simulink model "Sub3_2023"  (R2023b)
settings: Solver=FixedStepDiscrete  StartTime=0.0  StopTime=4.5  FixedStep=75e-6  RelTol=1e-3  EnableMultiTasking=on
undefined symbols (not defined in the file or in its folder): D1, D11, Delta
libraries: spsSeriesRLCBranchLib x41, spsLoadFlowBusLib x29, spsDistributedParametersLineLib x19, spsThreePhaseSeriesRLCLoadLib x15, spsThreePhaseTransformerTwoWindingsLib x13, spsThreePhaseParallelRLCLoadLib x11, spsThreePhaseVIMeasurementLib x11, spsSynchronousMachinepuStandardLib x7, spsExcitationSystemLib x7, spsHydraulicTurbineandGovernorLib x7, spsGenericPowerSystemStabilizerLib x7, spsMultiBandPowerSystemStabilizerLib x7
(part 2 of 5)

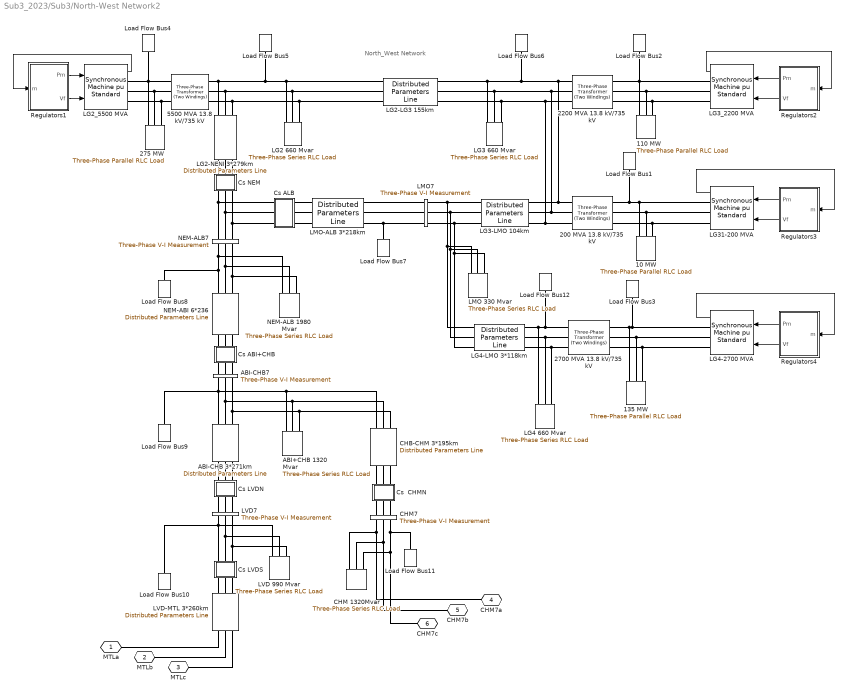
== system Sub3_2023/Sub3/North-West Network2 ==
  note: North_West Network
  10 MW : spsThreePhaseParallelRLCLoadLib/Three-Phase Parallel RLC Load  LConnTagsString=A|B|C  Configuration=Y (grounded)  NominalVoltage=(13800)*1  Vabc=[1e3 1e3 1e3]  Vabcp=[1e3 1e3 1e3]  NominalFrequency=60  UnbalancedPower=off  ActivePower=10000000  InductivePower=0  CapacitivePower=0  Pabc=[10e3 9e3 11e3]  QLabc=[100 90 110]  QCabc=[100 90 110]  Pabcp=[10e3 9e3 11e3]  QLabcp=[100 90 110]  QCabcp=[100 90 110]  Measurements=None  LoadType=constant PQ
  110 MW : spsThreePhaseParallelRLCLoadLib/Three-Phase Parallel RLC Load  LConnTagsString=A|B|C  Configuration=Y (grounded)  NominalVoltage=(13800)*1  Vabc=[1e3 1e3 1e3]  Vabcp=[1e3 1e3 1e3]  NominalFrequency=60  UnbalancedPower=off  ActivePower=110000000  InductivePower=0  CapacitivePower=0  Pabc=[10e3 9e3 11e3]  QLabc=[100 90 110]  QCabc=[100 90 110]  Pabcp=[10e3 9e3 11e3]  QLabcp=[100 90 110]  QCabcp=[100 90 110]  Measurements=None  LoadType=constant PQ
  135 MW : spsThreePhaseParallelRLCLoadLib/Three-Phase Parallel RLC Load  LConnTagsString=A|B|C  Configuration=Y (grounded)  NominalVoltage=(13800)*1  Vabc=[1e3 1e3 1e3]  Vabcp=[1e3 1e3 1e3]  NominalFrequency=60  UnbalancedPower=off  ActivePower=135000000  InductivePower=0  CapacitivePower=0  Pabc=[10e3 9e3 11e3]  QLabc=[100 90 110]  QCabc=[100 90 110]  Pabcp=[10e3 9e3 11e3]  QLabcp=[100 90 110]  QCabcp=[100 90 110]  Measurements=None  LoadType=constant PQ
  200 MVA 13.8 kV/735 kV : spsThreePhaseTransformerTwoWindingsLib/Three-Phase Transformer (Two Windings)  Winding1Connection=Delta (D1)  Winding2Connection=Yg  CoreType=Three single-phase transformers  SetSaturation=off  Hysteresis=off  DataFile='basic_model'  SetInitialFlux=off  Measurements=None  UNITS=pu  NominalPower=[ 200e6 60 ]  Winding1="[ 13.8e3 0.002  0.0]"  Winding2=[ 735e3 0.002 0.12]  Rm=500  Lm=500  L0=0.5  Saturation="[ 0,0  ;  0.005,1.2  ;  1.0,1.4 ]"  InitialFluxes=[ 0.8 , -0.8 , 0.7 ]  BreakLoop=off  DiscreteSolver=Trapezoidal iterative  DataType=off  TransfoNumber=0
  2200 MVA 13.8 kV/735 kV : spsThreePhaseTransformerTwoWindingsLib/Three-Phase Transformer (Two Windings)  Winding1Connection=Delta (D1)  Winding2Connection=Yg  CoreType=Three single-phase transformers  SetSaturation=off  Hysteresis=off  DataFile='basic_model'  SetInitialFlux=off  Measurements=None  UNITS=pu  NominalPower=[ 2200e6 60 ]  Winding1="[ 13.8e3 0.002  0.0]"  Winding2=[ 735e3 0.002 0.12]  Rm=500  Lm=500  L0=0.5  Saturation="[ 0,0  ;  0.005,1.2  ;  1.0,1.4 ]"  InitialFluxes=[ 0.8 , -0.8 , 0.7 ]  BreakLoop=off  DiscreteSolver=Trapezoidal iterative  DataType=off  TransfoNumber=0
  2700 MVA 13.8 kV/735 kV : spsThreePhaseTransformerTwoWindingsLib/Three-Phase Transformer (Two Windings)  Winding1Connection=Delta (D1)  Winding2Connection=Yg  CoreType=Three single-phase transformers  SetSaturation=off  Hysteresis=off  DataFile='basic_model'  SetInitialFlux=off  Measurements=None  UNITS=pu  NominalPower=[ 2700e6 60 ]  Winding1="[ 13.8e3 0.002  0.0]"  Winding2=[ 735e3 0.002 0.12]  Rm=500  Lm=500  L0=0.5  Saturation="[ 0,0  ;  0.005,1.2  ;  1.0,1.4 ]"  InitialFluxes=[ 0.8 , -0.8 , 0.7 ]  BreakLoop=off  DiscreteSolver=Trapezoidal iterative  DataType=off  TransfoNumber=0
  275 MW : spsThreePhaseParallelRLCLoadLib/Three-Phase Parallel RLC Load  LConnTagsString=A|B|C  Configuration=Y (grounded)  NominalVoltage=(13800)*1  Vabc=[1e3 1e3 1e3]  Vabcp=[1e3 1e3 1e3]  NominalFrequency=60  UnbalancedPower=off  ActivePower=275000000  InductivePower=0  CapacitivePower=0  Pabc=[10e3 9e3 11e3]  QLabc=[100 90 110]  QCabc=[100 90 110]  Pabcp=[10e3 9e3 11e3]  QLabcp=[100 90 110]  QCabcp=[100 90 110]  Measurements=None  LoadType=constant PQ
  5500 MVA 13.8 kV/735 kV : spsThreePhaseTransformerTwoWindingsLib/Three-Phase Transformer (Two Windings)  Winding1Connection=Delta (D1)  Winding2Connection=Yg  CoreType=Three single-phase transformers  SetSaturation=off  Hysteresis=off  DataFile='basic_model'  SetInitialFlux=off  Measurements=None  UNITS=pu  NominalPower=[ 5500e6 60 ]  Winding1="[ 13.8e3 0.002  0.0]"  Winding2=[ 735e3 0.002 0.12]  Rm=500  Lm=500  L0=0.5  Saturation="[ 0,0  ;  0.005,1.2  ;  1.0,1.4 ]"  InitialFluxes=[ 0.8 , -0.8 , 0.7 ]  BreakLoop=off  DiscreteSolver=Trapezoidal iterative  DataType=off  TransfoNumber=0
  ABI+CHB 1320 Mvar : spsThreePhaseSeriesRLCLoadLib/Three-Phase Series RLC Load  LConnTagsString=A|B|C  Configuration=Y (grounded)  NominalVoltage=735e3  Vabc=[1e3 1e3 1e3]  Vabcp=[1e3 1e3 1e3]  NominalFrequency=60  UnbalancedPower=off  ActivePower=4400000  InductivePower=1320e6  CapacitivePower=0  Pabc=[10e3 9e3 11e3]  QLabc=[100 90 110]  QCabc=[100 90 110]  Pabcp=[10e3 9e3 11e3]  QLabcp=[100 90 110]  QCabcp=[100 90 110]  Measurements=None  LoadType=constant Z
  ABI-CHB 3*271km : spsDistributedParametersLineLib/Distributed Parameters Line  Phases=3  Length=271  Frequency=60  Resistance="[0.01273  0.3864]/3"  Inductance="[0.9337e-3  4.1264e-3]/3"  Capacitance=[12.74e-9 7.751e-9]*3  x1=[-0.001575 2.82252813868878e-08 -103484.456536265 -819305.847115468;-0.0015 2.83466164414192e-08 -80280.8596539526 -821903.919579529;-0.001425 2.84452916444852e-08 -57013.087480771 -823844.97462583;-0.00135 2.85212281166381e-08 -33699.7399177867 -825127.460604666;-0.001275 2.8574365155424e-08 -10359.4532983355 -825750.352316369;-0.0012 2.86046602839071e-08 12989.1145095774 -825713.151830833;-0.001125 2.86120892846252e-08 36327.2990180915 -825015.888885559;-0.00105 2.85966462189488e-08 59636.4440395969 -823659.120861876;-0.000975 2.85583434318284e-08 82897.9166002052 -821643.932339383;-0.0009 2.84972115419259e-08 106093.121834664 -818971.934228952;-0.000825 2.84132994171387e-08 129203.517850807 -815645.262484989;-0.00075 2.83066741355355e-08 152210.630551661 -811666.576397987;-0.000675 2.8177420931735e-08 175096.068403352 -807039.056468727;-0.0006 2.80256431287707e-08 197841.537137021 -801766.401865838;-0.000525 2.78514620554959e-08 220428.85437298 -795852.827468734;-0.00045 2.76550169495957e-08 242839.964155428 -789303.060498309;-0.000375 2.74364648462819e-08 265056.951386106 -782122.336738063;-0.0003 2.71959804527619e-08 287062.056145353 -774316.396348701;-0.000225 2.69337560085805e-08 308837.687889115 -765891.479279537;-0.00015 2.66500011319461e-08 330366.439510553 -756854.320280369;-7.5e-05 2.63449426521655e-08 351631.101255022 -747212.143517828]  x2=[-0.001575 6.39967509370556e-08 -329701.158011639 -748762.18711566;-0.0015 6.42027184101767e-08 -308401.44101005 -757783.743021151;-0.001425 6.43573632125353e-08 -286855.192615217 -766199.538196952;-0.00135 6.44605617234425e-08 -265079.63656844 -774002.845185164;-0.001275 6.45122314475876e-08 -243092.179916044 -781187.426141576;-0.0012 6.45123310809837e-08 -220910.399094458 -787747.537822099;-0.001125 6.44608605439855e-08 -198552.025879879 -793677.936173828;-0.00105 6.43578609813526e-08 -176034.933213759 -798973.88052706;-0.000975 6.42034147293596e-08 -153377.120915453 -803631.137384908;-0.0009 6.3997645249977e-08 -130596.701293435 -807645.9838075;-0.000825 6.37407170321785e-08 -107711.884666601 -811015.210388034;-0.00075 6.34328354604501e-08 -84740.9648072106 -813736.123818332;-0.000675 6.30742466506096e-08 -61702.3043171338 -815806.549041831;-0.0006 6.26652372530649e-08 -38614.3199490629 -817224.830992284;-0.000525 6.22061342236703e-08 -15495.4678844435 -817989.835916801;-0.00045 6.16973045623632e-08 7635.77102011404 -818100.95228215;-0.000375 6.11391550197893e-08 30760.9060061493 -817558.09126361;-0.0003 6.0532131772153e-08 53861.451194581 -816361.686815971;-0.000225 5.98767200645508e-08 76918.9403630354 -814512.695326645;-0.00015 5.91734438230734e-08 99914.941707463 -812012.594851136;-7.5e-05 5.8422865235988e-08 122831.07257624 -808863.383931513]  x3=[-0.001575 1.3106440852015e-10 -747.841433918081 -1501.46113433883;-0.0015 1.39263740651287e-10 -705.09503694866 -1522.00231179706;-0.001425 1.47351747478955e-10 -661.784997795018 -1541.32682389466;-0.00135 1.55321963574244e-10 -617.945937839789 -1559.41922291233;-0.001275 1.63168017668359e-10 -573.612901356741 -1576.26504606312;-0.0012 1.70883637745703e-10 -528.82132749692 -1591.85082705374;-0.001125 1.78462656057641e-10 -483.607021959136 -1606.16410684936;-0.00105 1.85899014052897e-10 -438.006128367433 -1619.19344363309;-0.000975 1.93186767220669e-10 -392.055099378431 -1630.92842195248;-0.0009 2.00320089842582e-10 -345.790667541631 -1641.35966104539;-0.000825 2.07293279649674e-10 -299.249815935972 -1650.47882233891;-0.00075 2.14100762380708e-10 -252.46974860613 -1658.27861611503;-0.000675 2.20737096238147e-10 -205.487860822169 -1664.75280733794;-0.0006 2.27196976238244e-10 -158.341709186337 -1669.89622063824;-0.000525 2.33475238451766e-10 -111.06898161089 -1673.70474445002;-0.00045 2.3956686413196e-10 -63.7074671909556 -1676.17533429764;-0.000375 2.45466983726464e-10 -16.2950259965059 -1677.30601522935;-0.0003 2.51170880769947e-10 31.1304411924031 -1677.09588339614;-0.000225 2.56673995654386e-10 78.5310231829346 -1675.54510677417;-0.00015 2.61971929273943e-10 125.868828675099 -1672.65492503054;-7.5e-05 2.67060446541544e-10 173.106016551477 -1668.42764853232]  x4=[-0.001575 1.93458409580896e-10 -7080.29438162651 -14859.1258761624;-0.0015 1.8934224315803e-10 -6657.38891400317 -15053.3510061728;-0.001425 1.85074719443017e-10 -6229.16163154343 -15235.5427177129;-0.00135 1.80659249829019e-10 -5795.95485258481 -15405.5553695161;-0.001275 1.76099363974887e-10 -5358.11487599811 -15563.2530560699;-0.0012 1.71398706983604e-10 -4915.99170436145 -15708.5097162563;-0.001125 1.66561036488447e-10 -4469.93876417352 -15841.2092341238;-0.00105 1.6159021964919e-10 -4020.31262332986 -15961.2455317082;-0.000975 1.56490230060759e-10 -3567.47270608796 -16068.5226538298;-0.0009 1.51265144576798e-10 -3111.78100574897 -16162.9548447986;-0.000825 1.45919140050696e-10 -2653.60179528584 -16244.4666169659;-0.00075 1.40456489996676e-10 -2193.30133614902 -16312.9928110683;-0.000675 1.34881561173609e-10 -1731.24758548272 -16368.4786483147;-0.0006 1.29198810094297e-10 -1267.80990198557 -16410.8797741758;-0.000525 1.23412779463003e-10 -803.358750650903 -16440.1622938402;-0.00045 1.17528094544086e-10 -338.265406622771 -16456.3027993099;-0.000375 1.1154945946463e-10 127.098341595781 -16459.2883881117;-0.0003 1.05481653454042e-10 592.360489344731 -16449.1166736116;-0.000225 9.93295270236066e-11 1057.14911318192 -16425.7957869225;-0.00015 9.30979980890611e-11 1521.09266819295 -16389.3443704045;-7.5e-05 8.67920480392902e-11 1983.82028499853 -16339.7915627621]  x5=0.00153261764655846  V1=ones(3,3)  V2=ones(3,3)  I1=ones(3,3)  I2=ones(3,3)  nHarmo=1  Measurements=None  Decoupling=on  VsMag0=[674275.598206265 674275.04688371 674275.387112359]  VrMag0=[668005.988427177 668005.867389108 668005.726368268]  VsAngle0=[-3.17875639506823 -123.17875005978 116.821287344135]  VrAngle0=[-19.7452308032682 -139.745250763836 100.254768207184]  IsMag0=[1378.35069563023 1378.34088888681 1378.33344706177]  IrMag0=[13525.2461163751 13525.2482026069 13525.2572474099]  IsAngle0=[-22.4561903613039 -142.456782921015 97.5438663997709]  IrAngle0=[-21.4575985540813 -141.457549208484 98.5424184650414]
      settings: AttributesFormatString=\n  LibrarySourceBlock=sps_lib/Power Grid Elements/Distributed Parameters Line
  ABI-CHB7 : spsThreePhaseVIMeasurementLib/Three-Phase V-I Measurement  VoltageMeasurement=no  SetLabelV=on  LabelV=Vabc_ABI7  Vpu=on  VpuLL=off  CurrentMeasurement=no  SetLabelI=off  LabelI=A1  Ipu=off  Pbase=100e6  Vbase=500e3  OutputType=Magnitude  PhasorSimulation=off  PSBequivalent=0
  CHB-CHM 3*195km : spsDistributedParametersLineLib/Distributed Parameters Line  Phases=3  Length=195  Frequency=60  Resistance="[0.01273  0.3864]/3"  Inductance="[0.9337e-3  4.1264e-3]/3"  Capacitance=[12.74e-9 7.751e-9]*3  x1=[-0.001125 2.86120892846252e-08 0 0;-0.00105 2.85966462189488e-08 0 0;-0.000975 2.85583434318284e-08 0 0;-0.0009 2.84972115419259e-08 0 0;-0.000825 2.84132994171387e-08 0 0;-0.00075 2.83066741355355e-08 0 0;-0.000675 2.8177420931735e-08 175096.068403352 -807039.056468727;-0.0006 2.80256431287707e-08 197841.537137021 -801766.401865838;-0.000525 2.78514620554959e-08 220428.85437298 -795852.827468734;-0.00045 2.76550169495957e-08 242839.964155428 -789303.060498309;-0.000375 2.74364648462819e-08 265056.951386106 -782122.336738063;-0.0003 2.71959804527619e-08 287062.056145353 -774316.396348701;-0.000225 2.69337560085805e-08 308837.687889115 -765891.479279537;-0.00015 2.66500011319461e-08 330366.439510553 -756854.320280369;-7.5e-05 2.63449426521655e-08 351631.101255022 -747212.143517828]  x2=[-0.001125 1.92257365142825e-08 0 0;-0.00105 1.91619388673599e-08 0 0;-0.000975 1.90828234596942e-08 0 0;-0.0009 1.89884535349318e-08 0 0;-0.000825 1.88789045309467e-08 0 0;-0.00075 1.87542640195364e-08 0 0;-0.000675 1.86146316364188e-08 86661.6913680594 -814290.344127245;-0.0006 1.84601190015845e-08 109647.510746625 -811514.902082648;-0.000525 1.82908496300696e-08 132545.679582764 -808090.74744192;-0.00045 1.81069588332198e-08 155337.893430661 -804020.61742189;-0.000375 1.79085936105245e-08 178005.932543298 -799307.765622221;-0.0003 1.76959125321075e-08 200531.676437043 -793955.959424533;-0.000225 1.7469085611969e-08 222897.118376882 -787969.476980814;-0.00015 1.72282941720782e-08 245084.37977073 -781353.103793534;-7.5e-05 1.69737306974281e-08 267075.724461307 -774112.128890185]  x3=[-0.001125 1.04687394448767e-10 0 0;-0.00105 1.02659720732973e-10 0 0;-0.000975 1.00549982407171e-10 0 0;-0.0009 9.83598659638991e-11 0 0;-0.000825 9.60911221487322e-11 0 0;-0.00075 9.37455645607631e-11 0 0;-0.000675 9.13250682028394e-11 335.259499975967 -5255.1630322511;-0.0006 8.88315679827147e-11 483.692851575627 -5243.58412650791;-0.000525 8.62670571663132e-11 631.739546510486 -5227.81357984352;-0.00045 8.36335857843431e-11 779.281238517804 -5207.86399899163;-0.000375 8.09332589935339e-11 926.199985026453 -5183.75133134194;-0.0003 7.81682353938056e-11 1072.37834143841 -5155.49485219203;-0.000225 7.53407253027176e-11 1217.69945501215 -5123.11714933899;-0.00015 7.24529889885743e-11 1362.04715827299 -5086.64410502309;-7.5e-05 6.95073348636015e-11 1505.30606187552 -5046.10487523791]  x4=[-0.001125 8.04385281148192e-11 0 0;-0.00105 8.32616576275703e-11 0 0;-0.000975 8.601822904516e-11 0 0;-0.0009 8.8706038806574e-11 0 0;-0.000825 9.1322938317814e-11 0 0;-0.00075 9.38668356694505e-11 0 0;-0.000675 9.63356973088636e-11 265.942029612726 -12956.0177279482;-0.0006 9.87275496658336e-11 632.108856780154 -12943.3211843337;-0.000525 1.01040480730183e-10 997.770385799061 -12920.277947804;-0.00045 1.03272641580208e-10 1362.63431243796 -12886.9064387697;-0.000375 1.05422247860678e-10 1726.4089700565 -12843.2333339044;-0.0003 1.07487581209222e-10 2088.80356275932 -12789.2935448202;-0.000225 1.09466990629963e-10 2449.52839785384 -12725.1301901589;-0.00015 1.11358893813296e-10 2808.29511742615 -12650.7945611247;-7.5e-05 1.13161778400763e-10 3164.81692884995 -12566.3460804819]  x5=0.0011028060556417  V1=ones(3,3)  V2=ones(3,3)  I1=ones(3,3)  I2=ones(3,3)  nHarmo=1  Measurements=None  Decoupling=on  VsMag0=[674275.598206265 674275.04688371 674275.387112359]  VrMag0=[668620.174918554 668620.122023149 668619.982355037]  VsAngle0=[-3.17875639506823 -123.17875005978 116.821287344135]  VrAngle0=[-9.34509688682244 -129.345113323862 110.65489882013]  IsMag0=[4319.32992808175 4319.31639781994 4319.30396194623]  IrMag0=[10629.372791075 10629.3784873068 10629.3938662882]  IsAngle0=[-11.7695166369384 -131.769810740508 108.230491745392]  IrAngle0=[-14.2441447349322 -134.244031285624 105.755885398874]
      settings: AttributesFormatString=\n  LibrarySourceBlock=sps_lib/Power Grid Elements/Distributed Parameters Line
  CHM 1320Mvar : spsThreePhaseSeriesRLCLoadLib/Three-Phase Series RLC Load  LConnTagsString=A|B|C  Configuration=Y (grounded)  NominalVoltage=735e3  Vabc=[1e3 1e3 1e3]  Vabcp=[1e3 1e3 1e3]  NominalFrequency=60  UnbalancedPower=off  ActivePower=4400000  InductivePower=1320e6  CapacitivePower=0  Pabc=[10e3 9e3 11e3]  QLabc=[100 90 110]  QCabc=[100 90 110]  Pabcp=[10e3 9e3 11e3]  QLabcp=[100 90 110]  QCabcp=[100 90 110]  Measurements=None  LoadType=constant Z
  CHM7 : spsThreePhaseVIMeasurementLib/Three-Phase V-I Measurement  VoltageMeasurement=no  SetLabelV=on  LabelV=Vabc_CHM7  Vpu=on  VpuLL=off  CurrentMeasurement=no  SetLabelI=off  LabelI=A1  Ipu=off  Pbase=100e6  Vbase=735e3  OutputType=Magnitude  PhasorSimulation=off  PSBequivalent=0
  "Cs  CHMN " : Subsystem  mask{Xc=25/3}
      mask prompts: Xc "Condensator Reactance at  60Hz  (ohm):"
      mask help: Series Compensation
      mask init:
      | Cs=1/Xc/(2*pi*60);
      mask Display: disp('Cs')
  "Cs ABI+CHB " : Subsystem  mask{Xc=25/6}
      mask prompts: Xc "Condensator Reactance at  60Hz  (ohm):"
      mask help: Series Compensation
      mask init:
      | Cs=1/Xc/(2*pi*60);
      mask Display: disp('Cs')
  Cs ALB : Subsystem  mask{Xc=16/3}
      mask prompts: Xc "Reactance @ 60Hz du condensateur (ohm):"
      mask init:
      | Cs=1/Xc/(2*pi*60);
      mask Display: disp('Cs')
  "Cs LVDN " : Subsystem  mask{Xc=34/3}
      mask prompts: Xc "Condensator Reactance at  60Hz  (ohm):"
      mask help: Series Compensation
      mask init:
      | Cs=1/Xc/(2*pi*60);
      mask Display: disp('Cs')
  "Cs LVDS " : Subsystem  mask{Xc=34/3}
      mask prompts: Xc "Condensator Reactance at  60Hz  (ohm):"
      mask help: Series Compensation
      mask init:
      | Cs=1/Xc/(2*pi*60);
      mask Display: disp('Cs')
  "Cs NEM " : Subsystem  mask{Xc=16/3}
      mask prompts: Xc "Condensator Reactance at  60Hz  (ohm):"
      mask help: Series Compensation
      mask init:
      | Cs=1/Xc/(2*pi*60);
      mask Display: disp('Cs')
  LG2 660 Mvar : spsThreePhaseSeriesRLCLoadLib/Three-Phase Series RLC Load  LConnTagsString=A|B|C  Configuration=Y (grounded)  NominalVoltage=735e3  Vabc=[1e3 1e3 1e3]  Vabcp=[1e3 1e3 1e3]  NominalFrequency=60  UnbalancedPower=off  ActivePower=2200000  InductivePower=660e6  CapacitivePower=0  Pabc=[10e3 9e3 11e3]  QLabc=[100 90 110]  QCabc=[100 90 110]  Pabcp=[10e3 9e3 11e3]  QLabcp=[100 90 110]  QCabcp=[100 90 110]  Measurements=None  LoadType=constant Z
  LG2-LG3 155km : spsDistributedParametersLineLib/Distributed Parameters Line  Phases=3  Length=155  Frequency=60  Resistance="[0.01273  0.3864]"  Inductance="[0.9337e-3  4.1264e-3]"  Capacitance=[12.74e-9 7.751e-9]  x1=[-0.0009 5.26292056031291e-10 371984.24988172 -674633.962928139;-0.000825 5.67978956510661e-10 390907.83551166 -663848.049238456;-0.00075 6.09211823302567e-10 409518.935398982 -652531.465575427;-0.000675 6.49957695484177e-10 427802.672115196 -640693.258242884;-0.0006 6.90184001428704e-10 445744.429920922 -628342.890522636;-0.000525 7.29858584842658e-10 463329.866449487 -615490.235109674;-0.00045 7.689497304711e-10 480544.924171997 -602145.566220082;-0.000375 8.07426189450328e-10 497375.841634708 -588319.551377989;-0.0003 8.45257204287745e-10 513809.164459722 -574023.242888115;-0.000225 8.82412533448924e-10 529831.75610021 -559268.069000727;-0.00015 9.18862475532227e-10 545430.80834157 -544065.824776068;-7.5e-05 9.54577893011657e-10 560593.851540113 -528428.66265557]  x2=[-0.0009 -2.84133647185834e-10 375373.731714329 -666225.896356635;-0.000825 -3.30481312850429e-10 394058.262242269 -655347.523812927;-0.00075 -3.76564796810066e-10 412427.788624667 -643945.276485836;-0.000675 -4.22347260632767e-10 430467.626543196 -632028.269157416;-0.0006 -4.67792106517448e-10 448163.355227441 -619606.028100988;-0.000525 -5.12863006549638e-10 465500.828982646 -606688.483465986;-0.00045 -5.5752393174146e-10 482466.188497565 -593285.961339946;-0.000375 -6.0173918083265e-10 499045.871923379 -579409.175493991;-0.0003 -6.454734088296e-10 515226.625714835 -565069.218818404;-0.000225 -6.88691655259606e-10 530995.515224926 -550277.554455142;-0.00015 -7.31359372117733e-10 546339.93504465 -535046.006634378;-7.5e-05 -7.73442451483964e-10 561247.619079581 -519386.751222389]  x3=[-0.0009 1.24259718768771e-11 1272.11889165543 -2673.50704029682;-0.000825 1.22505792748699e-11 1347.19195646242 -2636.47471081189;-0.00075 1.20653937472306e-11 1421.18809663214 -2597.33482378256;-0.000675 1.18705633284365e-11 1494.04816078233 -2556.11866703565;-0.0006 1.16662437629433e-11 1565.71390569248 -2512.85918813624;-0.000525 1.14525983806856e-11 1636.12804286265 -2467.59096804986;-0.00045 1.12297979665129e-11 1705.23428430896 -2420.35019349904;-0.000375 1.09980206236675e-11 1772.97738755935 -2371.17462803613;-0.0003 1.07574516314109e-11 1839.30319981359 -2320.10358185576;-0.000225 1.05082832969147e-11 1904.15870123218 -2267.17788037083;-0.00015 1.02507148015331e-11 1967.49204731961 -2212.43983157731;-7.5e-05 9.98495204158025e-12 2029.25261036805 -2155.9331922339]  x4=[-0.0009 -1.18025559648927e-11 974.452643997273 -2530.47846704078;-0.000825 -1.16866166993846e-11 1045.60107405565 -2501.91852232173;-0.00075 -1.15613353312983e-11 1115.91366661366 -2471.35858221657;-0.000675 -1.14268120086425e-11 1185.33421486063 -2438.82307587384;-0.0006 -1.1283154267303e-11 1253.80722507246 -2404.3380116795;-0.000525 -1.11304769450804e-11 1321.27796097246 -2367.93095646624;-0.00045 -1.09689020898898e-11 1387.69248748669 -2329.63101347693;-0.000375 -1.07985588621984e-11 1452.99771385883 -2289.4687991;-0.0003 -1.06195834317761e-11 1517.14143609013 -2247.47641839511;-0.000225 -1.04321188688434e-11 1580.07237867045 -2203.6874394289;-0.00015 -1.02363150297038e-11 1641.74023556719 -2158.13686644117;-7.5e-05 -1.00323284369503e-11 1702.09571043908 -2110.86111186299]  x5=0.000876589428843401  V1=ones(3,3)  V2=ones(3,3)  I1=ones(3,3)  I2=ones(3,3)  nHarmo=1  Measurements=None  Decoupling=on  VsMag0=[629022.539261878 629021.416248132 629022.998971626]  VrMag0=[624373.329666333 624372.279031978 624373.793132847]  VsAngle0=[18.311762016023 -101.68813057419 138.311904308239]  VrAngle0=[18.8383509464139 -101.161544280644 138.838486827789]  IsMag0=[2426.2546778534 2426.24994282991 2426.25518358254]  IrMag0=[2222.110354709 2222.10693756313 2222.11326012476]  IsAngle0=[14.8862320606581 -105.113689591392 134.886368071059]  IrAngle0=[10.5010096554468 -109.498852970977 130.501154646759]
      settings: AttributesFormatString=\n  LibrarySourceBlock=sps_lib/Power Grid Elements/Distributed Parameters Line
  LG2-NENI 3*279km : spsDistributedParametersLineLib/Distributed Parameters Line  Phases=3  Length=279  Frequency=60  Resistance="[0.01273  0.3864]/3"  Inductance="[0.9337e-3  4.1264e-3]/3"  Capacitance=[12.74e-9 7.751e-9]*3  x1=[-0.00165 9.19274009253425e-11 168997.444323809 -751627.644710141;-0.001575 1.36275318057477e-10 190178.800706863 -746549.517209721;-0.0015 1.80514298785439e-10 211208.131066464 -740874.609447834;-0.001425 2.24608979144913e-10 232068.624877684 -734607.457858916;-0.00135 2.68524110523091e-10 252743.606580946 -727753.072308057;-0.001275 3.12224587835874e-10 273216.548912214 -720316.932086191;-0.0012 3.55675477590337e-10 293471.086114634 -712304.981530033;-0.001125 3.98842045810032e-10 313491.027021073 -703723.625270272;-0.00105 4.41689785800794e-10 333260.367997085 -694579.723111802;-0.000975 4.84184445734868e-10 352763.305733975 -684880.584550103;-0.0009 5.26292056031291e-10 371984.24988172 -674633.962928139;-0.000825 5.67978956510661e-10 390907.83551166 -663848.049238455;-0.00075 6.09211823302567e-10 409518.935398982 -652531.465575427;-0.000675 6.49957695484177e-10 427802.672115196 -640693.258242883;-0.0006 6.90184001428704e-10 445744.429920922 -628342.890522636;-0.000525 7.29858584842658e-10 463329.866449487 -615490.235109674;-0.00045 7.689497304711e-10 480544.924171997 -602145.566220082;-0.000375 8.07426189450328e-10 497375.841634708 -588319.551377989;-0.0003 8.45257204287745e-10 513809.164459722 -574023.242888115;-0.000225 8.82412533448924e-10 529831.75610021 -559268.069000727;-0.00015 9.18862475532227e-10 545430.80834157 -544065.824776068;-7.5e-05 9.54577893011657e-10 560593.851540113 -528428.66265557]  x2=[-0.00165 1.62069086814666e-08 -47534.306464813 -809002.98310623;-0.001575 1.62900091845941e-08 -24644.3461225884 -810023.426229766;-0.0015 1.63600877036248e-08 -1734.68546714459 -810396.349020148;-0.001425 1.64170882188631e-08 21176.36186932 -810121.453368603;-0.00135 1.6460965164969e-08 44070.4811461156 -809198.95902251;-0.001275 1.64916834673833e-08 66929.3711545839 -807629.603409733;-0.0012 1.6509218570365e-08 89734.7588478049 -805414.641049137;-0.001125 1.6513556456621e-08 112468.413947791 -802555.842547744;-0.00105 1.65046936585115e-08 135112.163518491 -799055.493185335;-0.000975 1.64826372608217e-08 157647.906492961 -794916.391087632;-0.0009 1.64474048950984e-08 180057.628143073 -790141.844989523;-0.000825 1.63990247255557e-08 202323.414480223 -784735.671590104;-0.00075 1.63375354265608e-08 224427.466575488 -778702.192501675;-0.000675 1.62629861517186e-08 246352.114787829 -772046.230795103;-0.0006 1.61754364945788e-08 268079.832888922 -764773.107144337;-0.000525 1.60749564409977e-08 289593.252073363 -756888.63557314;-0.00045 1.59616263131928e-08 310875.174843021 -748399.118807451;-0.000375 1.58355367055341e-08 331908.58875446 -739311.343237078;-0.0003 1.56967884121249e-08 352676.68001842 -729632.573490764;-0.000225 1.5545492346228e-08 373162.846940507 -719370.546628954;-0.00015 1.53817694516034e-08 393350.713192334 -708533.465958907;-7.5e-05 1.52057506058283e-08 413224.140902502 -697129.994477099]  x3=[-0.00165 1.1335104188753e-11 -1677.04894977027 -1941.35400834239;-0.001575 1.44183717100263e-11 -1621.49508617396 -1987.98793711353;-0.0015 1.74901134055631e-11 -1564.64502421547 -2033.03269874498;-0.001425 2.05478737720511e-11 -1506.5442089645 -2076.45228514349;-0.00135 2.35892084826388e-11 -1447.23908532377 -2118.21198735605;-0.001275 2.66116863408925e-11 -1386.77706090175 -2158.27842331564;-0.0012 2.96128912242577e-11 -1325.20646811563 -2196.61956452641;-0.001125 3.25904240154707e-11 -1262.57652555525 -2233.2047616667;-0.00105 3.55419045203759e-11 -1198.9372986384 -2268.00476908969;-0.000975 3.84649733706169e-11 -1134.33965958938 -2300.9917682019;-0.0009 4.13572939096793e-11 -1068.83524677246 -2332.13938970097;-0.000825 4.42165540607781e-11 -1002.476423413 -2361.42273465484;-0.00075 4.70404681750966e-11 -935.316235739068 -2388.81839440561;-0.000675 4.98267788588993e-11 -867.408370577103 -2414.30446928204;-0.0006 5.25732587780575e-11 -798.807112435492 -2437.86058610582;-0.000525 5.52777124385463e-11 -729.567300110359 -2459.46791447759;-0.00045 5.79379779414891e-11 -659.744282848271 -2479.10918182964;-0.000375 6.05519287113462e-11 -589.393876100901 -2496.76868723338;-0.0003 6.31174751958671e-11 -518.572316907004 -2512.43231395039;-0.000225 6.56325665364462e-11 -447.336218937394 -2526.08754071713;-0.00015 6.8095192207548e-11 -375.74252723884 -2537.72345175426;-7.5e-05 7.05033836238904e-11 -303.848472713064 -2547.33074549252]  x4=[-0.00165 3.99069334535873e-11 -141.249463963127 -15427.0315937081;-0.001575 3.77027265348956e-11 294.936850750288 -15424.8591939201;-0.0015 3.54683806334829e-11 730.887397457898 -15410.3563977008;-0.001425 3.32056818512763e-11 1166.25368396293 -15383.5347983636;-0.00135 3.09164389550618e-11 1600.68768511729 -15344.4158366845;-0.001275 2.86024819305839e-11 2033.8421210275 -15293.030783763;-0.0012 2.62656605196834e-11 2465.370734665 -15229.4207160241;-0.001125 2.39078427416415e-11 2894.92856865864 -15153.6364823829;-0.00105 2.15309133999142e-11 3322.17224104838 -15065.738663596;-0.000975 1.91367725754491e-11 3746.76021977958 -14965.797523835;-0.0009 1.67273341077895e-11 4168.35309571843 -14853.8929545178;-0.000825 1.4304524065181e-11 4586.61385397051 -14730.1144104449;-0.00075 1.18702792049014e-11 5001.20814328527 -14594.5608382907;-0.000675 9.42654542504671e-12 5411.80454333133 -14447.3405975066;-0.0006 6.97527620901023e-12 5818.07482962885 -14288.5713737005;-0.000525 4.51843106389757e-12 6219.69423592709 -14118.3800845608;-0.00045 2.05797395412674e-12 6616.34171381764 -13936.9027784;-0.000375 -4.04128268534962e-13 7007.70018937559 -13744.2845253999;-0.0003 -2.86590743724217e-12 7393.45681662356 -13540.6793016447;-0.000225 -5.32539564339389e-12 7773.303227616 -13326.2498660352;-0.00015 -7.78062680974957e-12 8146.93577894382 -13101.1676301812;-7.5e-05 -1.02296382620811e-11 8514.05579446225 -12865.6125213783]  x5=0.00157786097191812  V1=ones(3,3)  V2=ones(3,3)  I1=ones(3,3)  I2=ones(3,3)  nHarmo=1  Measurements=None  Decoupling=on  VsMag0=[629022.539261878 629021.416248132 629022.998971626]  VrMag0=[661687.482462878 661686.807299265 661687.362394953]  VsAngle0=[18.311762016023 -101.68813057419 138.311904308239]  VrAngle0=[2.27736225154843 -117.722616000131 122.277423755881]  IsMag0=[2108.4463150902 2108.42876135728 2108.41340422784]  IrMag0=[12679.519598142 12679.5310413668 12679.5487055201]  IsAngle0=[-35.1815546032546 -155.182311890524 84.8184798658946]  IrAngle0=[5.11533890202885 -114.884539075263 125.115355131987]
      settings: AttributesFormatString=\n  LibrarySourceBlock=sps_lib/Power Grid Elements/Distributed Parameters Line
  LG2_5500 MVA : spsSynchronousMachinepuStandardLib/Synchronous Machine pu Standard  PresetModel=No  MechanicalLoad=Mechanical power Pm  ShowDetailedParameters=on  RotorType=Salient-pole  Units=per unit standard parameters  MeasurementBus=off  NominalParameters="[5500E6  13800   60 ]"  Reactances1=[ 31 32 33 34 35 36 37 ]  Reactances2=[ 1.305, 0.296, 0.252, 0.474, 0.243, 0.18 ]  dAxisTimeConstants=Short-circuit  qAxisTimeConstants=Open-circuit  TimeConstants1=[]  TimeConstants2=[]  TimeConstants3=[]  TimeConstants4=[]  TimeConstants5=[ 1.01, 0.053, 0.1 ]  TimeConstants6=[]  TimeConstants7=[]  TimeConstants8=[]  StatorResistance=2.8544e-3  Mechanical="[ 4.1  0  32]"  PolePairs=32  InitialConditions=[0 -65.2434 0.985682 0.985682 0.985682 -1.22427 -121.224 118.776 1.47412]  SetSaturation=off  Saturation=[0.6404,0.7127,0.8441,0.9214,0.9956,1.082,1.19,1.316,1.457;0.7,0.7698,0.8872,0.9466,0.9969,1.046,1.1,1.151,1.201]  LoadFlowParameters=[2 4000000000 0 0 0]  TsPowergui=0  TsBlock=-1  IterativeModel=Trapezoidal non iterative  IterativeDiscreteModel=Trapezoidal non iterative  BusType=swing  Pref=0  Qref=0  Qmin=-Inf  Qmax=Inf  PLF=0  QLF=0
  LG3 660 Mvar : spsThreePhaseSeriesRLCLoadLib/Three-Phase Series RLC Load  LConnTagsString=A|B|C  Configuration=Y (grounded)  NominalVoltage=735e3  Vabc=[1e3 1e3 1e3]  Vabcp=[1e3 1e3 1e3]  NominalFrequency=60  UnbalancedPower=off  ActivePower=2200000  InductivePower=660e6  CapacitivePower=0  Pabc=[10e3 9e3 11e3]  QLabc=[100 90 110]  QCabc=[100 90 110]  Pabcp=[10e3 9e3 11e3]  QLabcp=[100 90 110]  QCabcp=[100 90 110]  Measurements=None  LoadType=constant Z
  LG3-LMO 104km : spsDistributedParametersLineLib/Distributed Parameters Line  Phases=3  Length=104  Frequency=60  Resistance="[0.01273  0.3864]"  Inductance="[0.9337e-3  4.1264e-3]"  Capacitance=[12.74e-9 7.751e-9]  x1=[-0.0006 -4.67792106517448e-10 0 0;-0.000525 -5.12863006549638e-10 0 0;-0.00045 -5.5752393174146e-10 0 0;-0.000375 -6.0173918083265e-10 499045.871923379 -579409.175493991;-0.0003 -6.454734088296e-10 515226.625714835 -565069.218818404;-0.000225 -6.88691655259606e-10 530995.515224926 -550277.554455142;-0.00015 -7.31359372117733e-10 546339.93504465 -535046.006634378;-7.5e-05 -7.73442451483964e-10 561247.619079581 -519386.751222389]  x2=[-0.0006 4.65360608460612e-09 0 0;-0.000525 4.57901919498695e-09 0 0;-0.00045 4.50077190748466e-09 0 0;-0.000375 4.41892677178365e-09 445735.713706768 -651849.764162704;-0.0003 4.33354921363311e-09 463985.717973717 -638987.984734801;-0.000225 4.24470748254673e-09 481864.819156937 -625615.408088745;-0.00015 4.152472597245e-09 499358.724976502 -611742.7240577;-7.5e-05 4.05691828888399e-09 516453.451071766 -597381.022253021]  x3=[-0.0006 1.25259114621196e-11 0 0;-0.000525 1.33034369985349e-11 0 0;-0.00045 1.40703279709631e-11 0 0;-0.000375 1.48259713384945e-11 -337.815764584562 -872.913223711159;-0.0003 1.55697630513829e-11 -313.002403558714 -882.114195189247;-0.000225 1.63011085339134e-11 -287.93883320056 -890.610018076502;-0.00015 1.70194231596972e-11 -262.645088944756 -898.393900942096;-7.5e-05 1.77241327190131e-11 -237.141390223455 -905.459621469165]  x4=[-0.0006 -7.12961610614154e-12 0 0;-0.000525 -7.92392068704507e-12 0 0;-0.00045 -8.71189100699143e-12 0 0;-0.000375 -9.4928971745632e-12 3507.69484614592 -3894.26054707398;-0.0003 -1.02663148653798e-11 3616.38515846578 -3793.5395268896;-0.000225 -1.10315258211729e-11 3722.18458782251 -3689.78600925053;-0.00015 -1.17879183440126e-11 3825.00855977106 -3583.08293313129;-7.5e-05 -1.25348877852893e-11 3924.77487840153 -3473.5155953383]  x5=0.000588163229675572  V1=ones(3,3)  V2=ones(3,3)  I1=ones(3,3)  I2=ones(3,3)  nHarmo=1  Measurements=None  Decoupling=on  VsMag0=[624373.329666333 624372.279031978 624373.793132847]  VrMag0=[644768.423999879 644767.634896167 644768.519320725]  VsAngle0=[18.8383509464139 -101.161544280644 138.838486827789]  VrAngle0=[12.4643674245556 -107.535582309775 132.464453284612]  IsMag0=[766.124869863951 766.121415585727 766.108315941418]  IrMag0=[4289.80561922833 4289.81652389775 4289.82131843341]  IsAngle0=[-43.0551695781816 -163.056449958927 76.9444139609184]  IrAngle0=[20.1104998668556 -99.8893421012274 140.110452750543]
      settings: AttributesFormatString=\n  LibrarySourceBlock=sps_lib/Power Grid Elements/Distributed Parameters Line
  LG31-200 MVA : spsSynchronousMachinepuStandardLib/Synchronous Machine pu Standard  PresetModel=No  MechanicalLoad=Mechanical power Pm  ShowDetailedParameters=on  RotorType=Salient-pole  Units=per unit standard parameters  MeasurementBus=off  NominalParameters="[200E6  13800   60 ]"  Reactances1=[ 31 32 33 34 35 36 37 ]  Reactances2=[ 1.305, 0.296, 0.252, 0.474, 0.243, 0.18 ]  dAxisTimeConstants=Short-circuit  qAxisTimeConstants=Open-circuit  TimeConstants1=[]  TimeConstants2=[]  TimeConstants3=[]  TimeConstants4=[]  TimeConstants5=[ 1.01, 0.053, 0.1 ]  TimeConstants6=[]  TimeConstants7=[]  TimeConstants8=[]  StatorResistance=2.8544e-3  Mechanical="[ 3.2  0  32]"  PolePairs=32  InitialConditions=[0 -67.6291 0.902477 0.902477 0.902477 -4.2812 -124.281 115.719 1.45511]  SetSaturation=off  Saturation=[0.6404,0.7127,0.8441,0.9214,0.9956,1.082,1.19,1.316,1.457;0.7,0.7698,0.8872,0.9466,0.9969,1.046,1.1,1.151,1.201]  LoadFlowParameters=[1 180000000 0 0 0]  TsPowergui=0  TsBlock=-1  IterativeModel=Trapezoidal non iterative  IterativeDiscreteModel=Trapezoidal non iterative  BusType=PV  Pref=180000000  Qref=0  Qmin=-Inf  Qmax=Inf  PLF=0  QLF=0
  LG3_2200 MVA : spsSynchronousMachinepuStandardLib/Synchronous Machine pu Standard  PresetModel=No  MechanicalLoad=Mechanical power Pm  ShowDetailedParameters=on  RotorType=Salient-pole  Units=per unit standard parameters  MeasurementBus=off  NominalParameters="[2200E6  13800   60 ]"  Reactances1=[ 31 32 33 34 35 36 37 ]  Reactances2=[ 1.305, 0.296, 0.252, 0.474, 0.243, 0.18 ]  dAxisTimeConstants=Short-circuit  qAxisTimeConstants=Open-circuit  TimeConstants1=[]  TimeConstants2=[]  TimeConstants3=[]  TimeConstants4=[]  TimeConstants5=[ 1.01, 0.053, 0.1 ]  TimeConstants6=[]  TimeConstants7=[]  TimeConstants8=[]  StatorResistance=2.8544e-3  Mechanical="[ 3.2  0  32]"  PolePairs=32  InitialConditions=[0 -70.0065 0.820496 0.820496 0.820496 -4.90643 -124.906 115.094 1.38903]  SetSaturation=off  Saturation=[0.6404,0.7127,0.8441,0.9214,0.9956,1.082,1.19,1.316,1.457;0.7,0.7698,0.8872,0.9466,0.9969,1.046,1.1,1.151,1.201]  LoadFlowParameters=[1 1800000000 0 0 0]  TsPowergui=0  TsBlock=-1  IterativeModel=Trapezoidal non iterative  IterativeDiscreteModel=Trapezoidal non iterative  BusType=PV  Pref=1800000000  Qref=0  Qmin=-Inf  Qmax=Inf  PLF=0  QLF=0
  LG4 660 Mvar : spsThreePhaseSeriesRLCLoadLib/Three-Phase Series RLC Load  LConnTagsString=A|B|C  Configuration=Y (grounded)  NominalVoltage=735e3  Vabc=[1e3 1e3 1e3]  Vabcp=[1e3 1e3 1e3]  NominalFrequency=60  UnbalancedPower=off  ActivePower=2200000  InductivePower=660e6  CapacitivePower=0  Pabc=[10e3 9e3 11e3]  QLabc=[100 90 110]  QCabc=[100 90 110]  Pabcp=[10e3 9e3 11e3]  QLabcp=[100 90 110]  QCabcp=[100 90 110]  Measurements=None  LoadType=constant Z
  LG4-2700 MVA : spsSynchronousMachinepuStandardLib/Synchronous Machine pu Standard  PresetModel=No  MechanicalLoad=Mechanical power Pm  ShowDetailedParameters=on  RotorType=Salient-pole  Units=per unit standard parameters  MeasurementBus=off  NominalParameters="[2700E6  13800   60 ]"  Reactances1=[ 31 32 33 34 35 36 37 ]  Reactances2=[ 1.305, 0.296, 0.252, 0.474, 0.243, 0.18 ]  dAxisTimeConstants=Short-circuit  qAxisTimeConstants=Open-circuit  TimeConstants1=[]  TimeConstants2=[]  TimeConstants3=[]  TimeConstants4=[]  TimeConstants5=[ 1.01, 0.053, 0.1 ]  TimeConstants6=[]  TimeConstants7=[]  TimeConstants8=[]  StatorResistance=2.8544e-3  Mechanical="[ 3.7  0  32]"  PolePairs=32  InitialConditions=[0 -69.506 0.926038 0.926038 0.926038 -2.40174 -122.402 117.598 1.38766]  SetSaturation=off  Saturation=[0.6404,0.7127,0.8441,0.9214,0.9956,1.082,1.19,1.316,1.457;0.7,0.7698,0.8872,0.9466,0.9969,1.046,1.1,1.151,1.201]  LoadFlowParameters=[1 2500000000 0 0 0]  TsPowergui=0  TsBlock=-1  IterativeModel=Trapezoidal non iterative  IterativeDiscreteModel=Trapezoidal non iterative  BusType=PV  Pref=2500000000  Qref=0  Qmin=-Inf  Qmax=Inf  PLF=0  QLF=0
  LG4-LMO 3*118km : spsDistributedParametersLineLib/Distributed Parameters Line  Phases=3  Length=118  Frequency=60  Resistance="[0.01273  0.3864]/3"  Inductance="[0.9337e-3  4.1264e-3]/3"  Capacitance=[12.74e-9 7.751e-9]*3  x1=[-0.000675 -5.49021082775681e-10 400494.989180275 -665247.597360457;-0.0006 -6.16600765132838e-10 419141.837998139 -653659.45092727;-0.000525 -6.83687546272655e-10 437453.631243793 -641548.779130337;-0.00045 -7.50227798048753e-10 455415.730749895 -628925.263055392;-0.000375 -8.1616832920196e-10 473013.77788893 -615798.99374804;-0.0003 -8.81456427880598e-10 490233.705051274 -602180.464147126;-0.000225 -9.46039903777523e-10 507061.746890627 -588080.560696844;-0.00015 -1.00986712985026e-09 523484.451327821 -573510.554644274;-7.5e-05 -1.07288708359089e-09 539488.690304204 -558482.093029328]  x2=[-0.000675 4.7244729527238e-09 369322.64221174 -697989.574610705;-0.0006 4.65360608460612e-09 388907.582416618 -687269.594638381;-0.000525 4.57901919498695e-09 408181.635850598 -676000.221867682;-0.00045 4.50077190748466e-09 427129.395130267 -664190.464862771;-0.000375 4.41892677178365e-09 445735.713706768 -651849.764162704;-0.0003 4.33354921363311e-09 463985.717973717 -638987.984734801;-0.000225 4.24470748254673e-09 481864.819156937 -625615.408088745;-0.00015 4.152472597245e-09 499358.724976502 -611742.7240577;-7.5e-05 4.05691828888399e-09 516453.451071766 -597381.022253021]  x3=[-0.000675 2.30755414381289e-11 1409.06764658949 -5515.47701855118;-0.0006 2.48646985501253e-11 1564.42956176252 -5473.43717855262;-0.000525 2.66339792025434e-11 1718.54089588045 -5427.02195661992;-0.00045 2.83819690595006e-11 1871.27845470077 -5376.26845637132;-0.000375 3.01072708046502e-11 2022.52014215593 -5321.21724937836;-0.0003 3.18085052581753e-11 2172.14505795504 -5261.9123427336;-0.000225 3.34843124792835e-11 2320.03359422976 -5198.40114387202;-0.00015 3.51333528533229e-11 2466.06753114695 -5130.73442267424;-7.5e-05 3.67543081626497e-11 2610.13013141185 -5058.96627088183]  x4=[-0.000675 -6.21909399594273e-12 5928.29142347596 -10182.4197288328;-0.0006 -8.70860350557629e-12 6213.78510946784 -10010.7531725401;-0.000525 -1.11911514908136e-11 6494.31159071731 -9831.08417333097;-0.00045 -1.36647534407795e-11 6769.64661864747 -9643.55635585427;-0.000375 -1.61274319959226e-11 7039.57009464974 -9448.31962697807;-0.0003 -1.85772185286861e-11 7303.86624602738 -9245.5300559562;-0.000225 -2.10121547171988e-11 7562.32379848085 -9035.34974966895;-0.00015 -2.34302941107273e-11 7814.73614499725 -8817.94672303731;-7.5e-05 -2.58297036856392e-11 8060.90151100881 -8593.49476471438]  x5=0.000667339049054976  V1=ones(3,3)  V2=ones(3,3)  I1=ones(3,3)  I2=ones(3,3)  nHarmo=1  Measurements=None  Decoupling=on  VsMag0=[634009.111289839 634008.470411781 634009.201310545]  VrMag0=[644768.423999879 644767.634896167 644768.519320725]  VsAngle0=[15.6289474446946 -104.371009723432 135.6290190178]  VrAngle0=[12.4643674245556 -107.535582309775 132.464453284612]  IsMag0=[4660.90997377898 4660.90842170641 4660.92192965187]  IrMag0=[9647.08196528224 9647.06470090362 9647.07193651076]  IsAngle0=[-1.08892209654313 -121.088741372855 118.911184788458]  IrAngle0=[14.7883279717914 -105.211681606025 134.788411982016]
      settings: AttributesFormatString=\n  LibrarySourceBlock=sps_lib/Power Grid Elements/Distributed Parameters Line
  LMO 330 Mvar : spsThreePhaseSeriesRLCLoadLib/Three-Phase Series RLC Load  LConnTagsString=A|B|C  Configuration=Y (grounded)  NominalVoltage=735e3  Vabc=[1e3 1e3 1e3]  Vabcp=[1e3 1e3 1e3]  NominalFrequency=60  UnbalancedPower=off  ActivePower=1100000  InductivePower=330e6  CapacitivePower=0  Pabc=[10e3 9e3 11e3]  QLabc=[100 90 110]  QCabc=[100 90 110]  Pabcp=[10e3 9e3 11e3]  QLabcp=[100 90 110]  QCabcp=[100 90 110]  Measurements=None  LoadType=constant Z
  LMO-ALB 3*218km : spsDistributedParametersLineLib/Distributed Parameters Line  Phases=3  Length=218  Frequency=60  Resistance="[0.01273  0.3864]/3"  Inductance="[0.9337e-3  4.1264e-3]/3"  Capacitance=[12.74e-9 7.751e-9]*3  x1=[-0.001275 5.1513334154814e-09 0 0;-0.0012 5.11200742750779e-09 0 0;-0.001125 5.06859497901296e-09 0 0;-0.00105 5.02113077324402e-09 0 0;-0.000975 4.96965275236082e-09 0 0;-0.0009 4.91420206710562e-09 0 0;-0.000825 4.85482304390779e-09 329282.961098489 -717747.524634782;-0.00075 4.79156314944995e-09 349442.471137504 -708151.592396683;-0.000675 4.7244729527238e-09 369322.64221174 -697989.574610705;-0.0006 4.65360608460612e-09 388907.582416618 -687269.594638381;-0.000525 4.57901919498695e-09 408181.635850598 -676000.221867682;-0.00045 4.50077190748466e-09 427129.395130267 -664190.464862771;-0.000375 4.41892677178365e-09 445735.713706768 -651849.764162704;-0.0003 4.33354921363311e-09 463985.717973717 -638987.984734801;-0.000225 4.24470748254673e-09 481864.819156937 -625615.408088745;-0.00015 4.152472597245e-09 499358.724976502 -611742.7240577;-7.5e-05 4.05691828888399e-09 516453.451071766 -597381.022253021]  x2=[-0.001275 1.67923283731231e-08 0 0;-0.0012 1.68076798761309e-08 0 0;-0.001125 1.68095955770118e-08 0 0;-0.00105 1.67980739443839e-08 0 0;-0.000975 1.6773124188464e-08 0 0;-0.0009 1.67347662537052e-08 0 0;-0.000825 1.66830308028538e-08 208359.206060502 -779372.311347925;-0.00075 1.66179591924374e-08 230309.218727131 -773170.335952805;-0.000675 1.6539603439706e-08 252075.125728158 -766350.300021026;-0.0006 1.64480261810492e-08 273639.527730558 -758917.655384964;-0.000525 1.63433006219266e-08 294985.186481314 -750878.343587016;-0.00045 1.62255104783477e-08 316095.038587422 -742238.791130029;-0.000375 1.6094749909951e-08 336952.2091561 -733005.904340047;-0.0003 1.59511234447343e-08 357540.02528432 -723187.063845501;-0.000225 1.57947458954962e-08 377842.029386873 -712790.118677251;-0.00015 1.56257422680569e-08 397841.992352312 -701823.379994185;-7.5e-05 1.54442476613305e-08 417523.926516251 -690295.614439409]  x3=[-0.001275 2.52140315525409e-11 0 0;-0.0012 2.81279817317481e-11 0 0;-0.001125 3.10194468327315e-11 0 0;-0.00105 3.38861154625302e-11 0 0;-0.000975 3.67256960501032e-11 0 0;-0.0009 3.95359186781757e-11 0 0;-0.000825 4.23145368977767e-11 -103.698287434644 -3735.86307130006;-0.00075 4.50593295240157e-11 1.95817417123465 -3737.30097845915;-0.000675 4.77681024116642e-11 107.613070442642 -3735.75134439868;-0.0006 5.04386902091212e-11 213.181942472072 -3731.21540787241;-0.000525 5.30689580893628e-11 318.580400118483 -3723.6967948386;-0.00045 5.56568034564901e-11 423.724189467484 -3713.20151556146;-0.000375 5.8200157626512e-11 528.529260182621 -3699.73795980667;-0.0003 6.06969874810195e-11 632.911832693937 -3683.3168901347;-0.000225 6.31452970924297e-11 736.788465170074 -3663.9514332974;-0.00015 6.55431293194997e-11 840.076120220395 -3641.65706974465;-7.5e-05 6.78885673718351e-11 942.692231273807 -3616.45162124958]  x4=[-0.001275 5.95793005777818e-11 0 0;-0.0012 5.721772520544e-11 0 0;-0.001125 5.48104108590294e-11 0 0;-0.00105 5.23592819088056e-11 0 0;-0.000975 4.98662977497478e-11 0 0;-0.0009 4.73334512352487e-11 0 0;-0.000825 4.47627670840583e-11 3660.66083936772 -13572.4875623724;-0.00075 4.21563002617542e-11 4042.89932356784 -13463.5735253596;-0.000675 3.95161343380338e-11 4421.90597590715 -13343.8969136702;-0.0006 3.68443798211408e-11 4797.37782426674 -13213.5533949565;-0.000525 3.41431724707567e-11 5169.01472219595 -13072.647163833;-0.00045 3.14146715907075e-11 5536.51958884482 -12921.290858585;-0.000375 2.86610583028493e-11 5899.59864644595 -12759.6054711269;-0.0003 2.58845338035126e-11 6257.961655156 -12587.7202502838;-0.000225 2.30873176039001e-11 6611.32214506895 -12405.7725984711;-0.00015 2.02716457558429e-11 6959.39764521575 -12213.907961858;-7.5e-05 1.7439769064335e-11 7301.90990936732 -12012.2797140992]  x5=0.00123288061605072  V1=ones(3,3)  V2=ones(3,3)  I1=ones(3,3)  I2=ones(3,3)  nHarmo=1  Measurements=None  Decoupling=on  VsMag0=[644768.423999879 644767.634896167 644768.519320725]  VrMag0=[658703.501124779 658702.724611139 658703.398472697]  VsAngle0=[12.4643674245556 -107.535582309775 132.464453284612]  VrAngle0=[2.78756158795561 -117.212409726232 122.787634425005]  IsMag0=[3067.18219524842 3067.16950451142 3067.1745038963]  IrMag0=[11536.865176044 11536.8607652593 11536.8706203299]  IsAngle0=[-13.7698967097776 -133.769925743281 106.230294079488]  IrAngle0=[2.91418185480181 -117.085774277238 122.91422275938]
      settings: AttributesFormatString=\n  LibrarySourceBlock=sps_lib/Power Grid Elements/Distributed Parameters Line
  LMO7 : spsThreePhaseVIMeasurementLib/Three-Phase V-I Measurement  VoltageMeasurement=no  SetLabelV=on  LabelV=Vabc_LMO7  Vpu=on  VpuLL=off  CurrentMeasurement=no  SetLabelI=off  LabelI=A1  Ipu=off  Pbase=100e6  Vbase=735e3  OutputType=Magnitude  PhasorSimulation=off  PSBequivalent=0
  LVD 990 Mvar : spsThreePhaseSeriesRLCLoadLib/Three-Phase Series RLC Load  LConnTagsString=A|B|C  Configuration=Y (grounded)  NominalVoltage=735e3  Vabc=[1e3 1e3 1e3]  Vabcp=[1e3 1e3 1e3]  NominalFrequency=60  UnbalancedPower=off  ActivePower=3300000  InductivePower=990e6  CapacitivePower=0  Pabc=[10e3 9e3 11e3]  QLabc=[100 90 110]  QCabc=[100 90 110]  Pabcp=[10e3 9e3 11e3]  QLabcp=[100 90 110]  QCabcp=[100 90 110]  Measurements=None  LoadType=constant Z
  LVD-MTL 3*260km : spsDistributedParametersLineLib/Distributed Parameters Line  Phases=3  Length=260  Frequency=60  Resistance="[0.01273  0.3864]/3"  Inductance="[0.9337e-3  4.1264e-3]/3"  Capacitance=[12.74e-9 7.751e-9]*3  x1=[-0.0015 5.83226266055962e-08 -149994.752694971 -815900.545010702;-0.001425 5.85173753833575e-08 -126868.831368553 -819814.85417162;-0.00135 5.86653462665833e-08 -103641.493039497 -823073.815881701;-0.001275 5.87664209696134e-08 -80331.3052866728 -825674.824976819;-0.0012 5.88205186948767e-08 -56956.901917513 -827615.802250098;-0.001125 5.88275961974796e-08 -33536.9680724301 -828895.196114005;-0.00105 5.87876478197745e-08 -10090.2252882029 -829511.98384066;-0.000975 5.87007054958835e-08 13364.5834677339 -829465.672379392;-0.0009 5.856683872617e-08 36808.7087801317 -828756.298750874;-0.000825 5.83861545216815e-08 60223.4097739227 -827384.430017531;-0.00075 5.81587973186065e-08 83589.9690953896 -825351.162830238;-0.000675 5.78849488628144e-08 106889.707874531 -822658.122551676;-0.0006 5.75648280645708e-08 130104.000656665 -819307.461957037;-0.000525 5.71986908235438e-08 153214.290291332 -815301.859513133;-0.00045 5.67868298242418e-08 176202.102766597 -810644.517237272;-0.000375 5.63295743020459e-08 199049.061976893 -805339.158137609;-0.0003 5.58272897800243e-08 221736.904412598 -799390.023237032;-0.000225 5.52803777767387e-08 244247.493759604 -792801.868182958;-0.00015 5.46892754852766e-08 266562.83539721 -785579.959445733;-7.5e-05 5.40544554237655e-08 288665.090782748 -777730.070108704]  x2=[-0.0015 8.96214664117817e-08 -353353.509255454 -707507.47627998;-0.001425 8.98036943913653e-08 -333210.629182348 -717214.190537918;-0.00135 8.9914134671695e-08 -312801.385630568 -726347.574745686;-0.001275 8.99526989685005e-08 -292142.093437137 -734900.327815692;-0.0012 8.99193564540731e-08 -271249.267324136 -742865.612807995;-0.001125 8.98141337819085e-08 -250139.608697089 -750237.062395643;-0.00105 8.96371150654011e-08 -228829.992294114 -757008.783954625;-0.000975 8.93884418106042e-08 -207337.452696515 -763175.364274336;-0.0009 8.90683128031129e-08 -185679.1707116 -768731.873884821;-0.000825 8.86769839491577e-08 -163872.459638605 -773673.870997315;-0.00075 8.82147680710369e-08 -141934.751428708 -777997.40505494;-0.000675 8.76820346570513e-08 -119883.582750192 -781699.019890724;-0.0006 8.7079209566141e-08 -97736.5809699071 -784775.756490404;-0.000525 8.64067746874602e-08 -75511.4500622143 -787225.155357816;-0.00045 8.56652675551621e-08 -53225.9564567056 -789045.258480985;-0.000375 8.4855280918703e-08 -30897.9148359899 -790234.610897321;-0.0003 8.39774622690068e-08 -8545.17389490828 -790792.261856701;-0.000225 8.30325133208711e-08 13814.3979274394 -790717.76558148;-0.00015 8.20211894520267e-08 36162.9267314513 -790011.18162284;-7.5e-05 8.09442990993006e-08 58482.5474451453 -788673.074813188]  x3=[-0.0015 2.58388491658684e-10 176.513539924813 -1804.5571384245;-0.001425 2.66925459819509e-10 227.459268206878 -1798.84517601313;-0.00135 2.7524905185185e-10 278.223169030182 -1791.69524429131;-0.001275 2.83352614003593e-10 328.764662509121 -1783.11305880506;-0.0012 2.91229668411142e-10 379.043346547118 -1773.10548002214;-0.001125 2.98873918277727e-10 429.019029133443 -1761.68050784792;-0.00105 3.06279252906964e-10 478.65176047209 -1748.84727523034;-0.000975 3.13439752587657e-10 527.901864917033 -1734.61604085921;-0.0009 3.20349693325921e-10 576.729972688331 -1718.99818096552;-0.000825 3.27003551420855e-10 625.097051343726 -1702.00618022753;-0.00075 3.33396007880105e-10 672.964436980582 -1683.65362179063;-0.000675 3.39521952671785e-10 720.293865143218 -1663.95517640923;-0.0006 3.4537648880936e-10 767.047501410924 -1642.92659071918;-0.000525 3.50954936266218e-10 813.187971642222 -1620.58467465013;-0.00045 3.56252835716816e-10 858.678391851183 -1596.94728798794;-0.000375 3.61265952101392e-10 903.482397691917 -1572.03332609785;-0.0003 3.65990278011414e-10 947.564173527681 -1545.86270481979;-0.000225 3.70422036893031e-10 990.888481061345 -1518.45634454799;-0.00015 3.74557686066004e-10 1033.42068750435 -1489.83615350752;-7.5e-05 3.78393919555661e-10 1075.12679326163 -1460.02501024119]  x4=[-0.0015 2.70359912182284e-10 -8566.49009753185 -13975.6180438591;-0.001425 2.67569555553607e-10 -8167.9678666522 -14212.2119177596;-0.00135 2.64565307916171e-10 -7762.91628723406 -14437.4447669072;-0.001275 2.61349570819573e-10 -7351.6591513125 -14651.1365436084;-0.0012 2.57924914874843e-10 -6934.52521154954 -14853.1164259265;-0.001125 2.54294077699547e-10 -6511.84791843426 -15043.2229542341;-0.00105 2.50459961729367e-10 -6083.9651537276 -15221.3041602811;-0.000975 2.46425631897946e-10 -5651.21896036484 -15387.2176886761;-0.0009 2.42194313186825e-10 -5213.95526903171 -15540.8309106831;-0.000825 2.3776938804744e-10 -4772.52362163271 -15682.0210302428;-0.00075 2.33154393697243e-10 -4327.27689187264 -15810.6751821339;-0.000675 2.28353019292107e-10 -3878.57100317475 -15926.6905221959;-0.0006 2.23369102977266e-10 -3426.76464416106 -16029.9743095409;-0.000525 2.18206628819168e-10 -2972.21898192209 -16120.4439806898;-0.00045 2.12869723620665e-10 -2515.29737330543 -16198.0272155715;-0.000375 2.07362653622115e-10 -2056.3650744539 -16262.6619953352;-0.0003 2.01689821091015e-10 -1595.78894882529 -16314.2966519269;-0.000225 1.95855760802893e-10 -1133.93717392739 -16352.8899093922;-0.00015 1.89865136416278e-10 -671.178947002458 -16378.4109168715;-7.5e-05 1.83722736744647e-10 -207.88418989668 -16390.839273262]  x5=0.00147040807418893  V1=ones(3,3)  V2=ones(3,3)  I1=ones(3,3)  I2=ones(3,3)  nHarmo=1  Measurements=None  Decoupling=on  VsMag0=[677344.070713929 677343.614711415 677343.797959389]  VrMag0=[645717.103800377 645717.117585074 645716.873803133]  VsAngle0=[-8.01690098277304 -128.016905354065 111.983130236572]  VrAngle0=[-24.1390927893337 -144.139117060795 95.8608940156664]  IsMag0=[1489.54148607982 1489.52649322814 1489.52592422187]  IrMag0=[13466.1974570838 13466.1988034392 13466.2083731064]  IsAngle0=[7.9869385974373 -112.013419640768 127.987258926251]  IrAngle0=[-29.1066680799827 -149.106617756854 90.8933521206026]
      settings: AttributesFormatString=\n  LibrarySourceBlock=sps_lib/Power Grid Elements/Distributed Parameters Line
  LVD7 : spsThreePhaseVIMeasurementLib/Three-Phase V-I Measurement  VoltageMeasurement=no  SetLabelV=on  LabelV=Vabc_LVD7  Vpu=on  VpuLL=off  CurrentMeasurement=no  SetLabelI=off  LabelI=A1  Ipu=off  Pbase=100e6  Vbase=735e3  OutputType=Magnitude  PhasorSimulation=off  PSBequivalent=0
  Load Flow Bus1 : spsLoadFlowBusLib/Load Flow Bus  LConnTagsString=a  Phases=single  Connectors=on one side  ID=LG31_13.8  Vbase=13.8e3  Vref=1  Vangle=0  VLF=1  VLFb=1  VLFc=1  angleLF=-0.0351  angleLFb=0  angleLFc=0
      settings: AttributesFormatString=%<ID>\n%<Vbase>V\n%<VLF>pu\n%<angleLF>deg.
  Load Flow Bus10 : spsLoadFlowBusLib/Load Flow Bus  LConnTagsString=a  Phases=single  Connectors=on one side  ID=LVD7  Vbase=735e3  Vref=1  Vangle=0  VLF=1.05  VLFb=1  VLFc=1  angleLF=-12.02  angleLFb=0  angleLFc=0
      settings: AttributesFormatString=%<ID>\n%<Vbase>V\n%<VLF>pu\n%<angleLF>deg.
  Load Flow Bus11 : spsLoadFlowBusLib/Load Flow Bus  LConnTagsString=a  Phases=single  Connectors=on one side  ID=CHM7  Vbase=735e3  Vref=1  Vangle=0  VLF=1.047  VLFb=1  VLFc=1  angleLF=-4.064  angleLFb=0  angleLFc=0
      settings: AttributesFormatString=%<ID>\n%<Vbase>V\n%<VLF>pu\n%<angleLF>deg.
  Load Flow Bus12 : spsLoadFlowBusLib/Load Flow Bus  LConnTagsString=a  Phases=single  Connectors=on one side  ID=LG47  Vbase=735e3  Vref=1  Vangle=0  VLF=1.004  VLFb=1  VLFc=1  angleLF=20.71  angleLFb=0  angleLFc=0
      settings: AttributesFormatString=%<ID>\n%<Vbase>V\n%<VLF>pu\n%<angleLF>deg.
  Load Flow Bus2 : spsLoadFlowBusLib/Load Flow Bus  LConnTagsString=a  Phases=single  Connectors=on one side  ID=LG3_13.8  Vbase=13.8e3  Vref=1  Vangle=0  VLF=1  VLFb=1  VLFc=1  angleLF=-0.6025  angleLFb=0  angleLFc=0
      settings: AttributesFormatString=%<ID>\n%<Vbase>V\n%<VLF>pu\n%<angleLF>deg.
  Load Flow Bus3 : spsLoadFlowBusLib/Load Flow Bus  LConnTagsString=a  Phases=single  Connectors=on one side  ID=LG4_13.8  Vbase=13.8e3  Vref=1  Vangle=0  VLF=1  VLFb=1  VLFc=1  angleLF=-3.293  angleLFb=0  angleLFc=0
      settings: AttributesFormatString=%<ID>\n%<Vbase>V\n%<VLF>pu\n%<angleLF>deg.
  Load Flow Bus4 : spsLoadFlowBusLib/Load Flow Bus  LConnTagsString=a  Phases=single  Connectors=on one side  ID=LG2_13.8  Vbase=13.8e3  Vref=1  Vangle=0  VLF=1  VLFb=1  VLFc=1  angleLF=0  angleLFb=0  angleLFc=0
      settings: AttributesFormatString=%<ID>\n%<Vbase>V\n%<VLF>pu\n%<angleLF>deg.
  Load Flow Bus5 : spsLoadFlowBusLib/Load Flow Bus  LConnTagsString=a  Phases=single  Connectors=on one side  ID=LG27  Vbase=735e3  Vref=1  Vangle=0  VLF=1  VLFb=1  VLFc=1  angleLF=23.57  angleLFb=0  angleLFc=0
      settings: AttributesFormatString=%<ID>\n%<Vbase>V\n%<VLF>pu\n%<angleLF>deg.
  Load Flow Bus6 : spsLoadFlowBusLib/Load Flow Bus  LConnTagsString=a  Phases=single  Connectors=on one side  ID=LG37  Vbase=735e3  Vref=1  Vangle=0  VLF=0.994  VLFb=1  VLFc=1  angleLF=24.1  angleLFb=0  angleLFc=0
      settings: AttributesFormatString=%<ID>\n%<Vbase>V\n%<VLF>pu\n%<angleLF>deg.
  Load Flow Bus7 : spsLoadFlowBusLib/Load Flow Bus  LConnTagsString=a  Phases=single  Connectors=on one side  ID=LMO7  Vbase=735e3  Vref=1  Vangle=0  VLF=1.016  VLFb=1  VLFc=1  angleLF=17.31  angleLFb=0  angleLFc=0
      settings: AttributesFormatString=%<ID>\n%<Vbase>V\n%<VLF>pu\n%<angleLF>deg.
  Load Flow Bus8 : spsLoadFlowBusLib/Load Flow Bus  LConnTagsString=a  Phases=single  Connectors=on one side  ID=NEM_ALB7  Vbase=735e3  Vref=1  Vangle=0  VLF=1.028  VLFb=1  VLFc=1  angleLF=8.928  angleLFb=0  angleLFc=0
      settings: AttributesFormatString=%<ID>\n%<Vbase>V\n%<VLF>pu\n%<angleLF>deg.
  Load Flow Bus9 : spsLoadFlowBusLib/Load Flow Bus  LConnTagsString=a  Phases=single  Connectors=on one side  ID=ABI_CHB7  Vbase=735e3  Vref=1  Vangle=0  VLF=1.046  VLFb=1  VLFc=1  angleLF=0.1334  angleLFb=0  angleLFc=0
      settings: AttributesFormatString=%<ID>\n%<Vbase>V\n%<VLF>pu\n%<angleLF>deg.
  NEM-ABI 6*236 : spsDistributedParametersLineLib/Distributed Parameters Line  Phases=3  Length=236  Frequency=60  Resistance="[0.01273  0.3864]/6"  Inductance="[0.9337e-3  4.1264e-3]/6"  Capacitance=[12.74e-9 7.751e-9]*6  x1=[-0.00135 1.62257836144723e-08 0 0;-0.001275 1.62651346738051e-08 0 0;-0.0012 1.62914836333445e-08 0 0;-0.001125 1.63048094301356e-08 0 0;-0.00105 1.63051014117401e-08 0 0;-0.000975 1.62923593447526e-08 0 0;-0.0009 1.62665934149862e-08 0 0;-0.000825 1.62278242193312e-08 235173.136251842 -772031.417007247;-0.00075 1.61760827492893e-08 256904.899781818 -765074.329412228;-0.000675 1.61114103661999e-08 278431.297465686 -757505.653104307;-0.0006 1.60338587681767e-08 299735.121430501 -749331.438367519;-0.000525 1.59434899487804e-08 320799.341725346 -740558.219544056;-0.00045 1.58403761474627e-08 341607.11993481 -731193.009810809;-0.000375 1.57245997918185e-08 362141.822639362 -721243.295573149;-0.0003 1.55962534316952e-08 382387.034711852 -710717.030480399;-0.000225 1.54554396652094e-08 402326.572439512 -699622.629067819;-0.00015 1.53022710567312e-08 421944.496460966 -687968.960030147;-7.5e-05 1.5136870046903e-08 441225.124507917 -675765.339132105]  x2=[-0.00135 2.94289926409663e-08 0 0;-0.001275 2.94762998726434e-08 0 0;-0.0012 2.95000442012047e-08 0 0;-0.001125 2.95002066457975e-08 0 0;-0.00105 2.94767870765658e-08 0 0;-0.000975 2.94298042147552e-08 0 0;-0.0009 2.93592956177464e-08 0 0;-0.000825 2.9265317649033e-08 81706.5138318558 -820341.457427416;-0.00075 2.91479454331654e-08 104865.377019272 -817703.667465278;-0.000675 2.9007272795697e-08 127940.412428793 -814412.217702655;-0.0006 2.88434121881819e-08 150913.174230172 -810469.739274124;-0.000525 2.86564945982825e-08 173765.298349121 -805879.383736621;-0.00045 2.84466694450604e-08 196478.517147267 -800644.820550126;-0.000375 2.82141044595325e-08 219034.674025028 -794770.234144361;-0.0003 2.795898555059e-08 241415.737935717 -788260.320573812;-0.000225 2.76815166563851e-08 263603.817799284 -781120.283763785;-0.00015 2.73819195813066e-08 285581.176804176 -773355.831350457;-7.5e-05 2.70604338186721e-08 307330.24658587 -764973.170118289]  x3=[-0.00135 1.59850883493891e-10 0 0;-0.001275 1.66708043820479e-10 0 0;-0.0012 1.73431940287557e-10 0 0;-0.001125 1.80017197915166e-10 0 0;-0.00105 1.86458552549117e-10 0 0;-0.000975 1.92750855069072e-10 0 0;-0.0009 1.98889075504671e-10 0 0;-0.000825 2.04868307056417e-10 -1379.76964293978 -6710.39772289979;-0.00075 2.10683770018093e-10 -1189.51028635564 -6746.7212182112;-0.000675 2.16330815597585e-10 -998.300053448707 -6777.65148780907;-0.0006 2.21804929633062e-10 -806.291794753548 -6803.16380650912;-0.000525 2.27101736201519e-10 -613.638998734341 -6823.23778015415;-0.00045 2.32217001116829e-10 -420.495669088537 -6837.85736191676;-0.000375 2.37146635314487e-10 -227.016201638664 -6847.01086512699;-0.0003 2.41886698120338e-10 -33.3552609106645 -6850.69097261441;-0.000225 2.46433400400703e-10 160.332343502554 -6848.89474255741;-0.00015 2.50783107591346e-10 353.891780693544 -6841.62361083481;-7.5e-05 2.5493234260289e-10 547.168322209773 -6828.88338987806]  x4=[-0.00135 1.66714476329562e-10 0 0;-0.001275 1.62860627074303e-10 0 0;-0.0012 1.58876589525613e-10 0 0;-0.001125 1.54765548462148e-10 0 0;-0.00105 1.50530790187236e-10 0 0;-0.000975 1.46175699901846e-10 0 0;-0.0009 1.41703758998518e-10 0 0;-0.000825 1.37118542278386e-10 2916.74328192214 -29367.011437799;-0.00075 1.32423715093541e-10 3745.79818278 -29272.8158501738;-0.000675 1.27623030417001e-10 4571.8587498832 -29155.2200214471;-0.0006 1.22720325842644e-10 5394.26464305352 -29014.317955925;-0.000525 1.17719520517492e-10 6212.3584436032 -28850.2222885629;-0.00045 1.12624612008808e-10 7025.48617986533 -28663.0641949266;-0.000375 1.07439673108498e-10 7832.99784996883 -28452.9932863324;-0.0003 1.02168848577387e-10 8634.24794143994 -28220.1774902505;-0.000225 9.68163518319589e-11 9428.59594721509 -27964.8029160661;-0.00015 9.13864615762165e-11 10215.4068776524 -27687.0737063064;-7.5e-05 8.58835183813497e-11 10994.0517681327 -27387.2118734524]  x5=0.00133467809810995  V1=ones(3,3)  V2=ones(3,3)  I1=ones(3,3)  I2=ones(3,3)  nHarmo=1  Measurements=None  Decoupling=on  VsMag0=[658958.583852788 658957.792322798 658958.516680612]  VrMag0=[673120.404843083 673119.992372496 673120.175209564]  VsAngle0=[4.76158286038345 -115.238384148901 124.761658957968]  VrAngle0=[-6.49205363089091 -126.492055930664 113.507975624827]  IsMag0=[5624.79821722641 5624.77239180783 5624.75565924746]  IrMag0=[24230.0809184606 24230.088493199 24230.1137544036]  IsAngle0=[-23.7987124057237 -143.799061097522 96.2013410714627]  IrAngle0=[-6.50799783402431 -126.507918517815 113.492026312171]
      settings: AttributesFormatString=\n  LibrarySourceBlock=sps_lib/Power Grid Elements/Distributed Parameters Line
  NEM-ALB 1980 Mvar : spsThreePhaseSeriesRLCLoadLib/Three-Phase Series RLC Load  LConnTagsString=A|B|C  Configuration=Y (grounded)  NominalVoltage=735e3  Vabc=[1e3 1e3 1e3]  Vabcp=[1e3 1e3 1e3]  NominalFrequency=60  UnbalancedPower=off  ActivePower=6600000  InductivePower=1980e6  CapacitivePower=0  Pabc=[10e3 9e3 11e3]  QLabc=[100 90 110]  QCabc=[100 90 110]  Pabcp=[10e3 9e3 11e3]  QLabcp=[100 90 110]  QCabcp=[100 90 110]  Measurements=None  LoadType=constant Z
  NEM-ALB7 : spsThreePhaseVIMeasurementLib/Three-Phase V-I Measurement  VoltageMeasurement=no  SetLabelV=on  LabelV=Vabc_NEM7  Vpu=on  VpuLL=off  CurrentMeasurement=no  SetLabelI=off  LabelI=A1  Ipu=off  Pbase=100e6  Vbase=735e3  OutputType=Magnitude  PhasorSimulation=off  PSBequivalent=0
  Regulators1 : Subsystem
  Regulators2 : Subsystem
  Regulators3 : Subsystem
  Regulators4 : Subsystem
  MTLa : PMIOPort  Side=Right
  MTLb : PMIOPort  Port=2  Side=Right
  MTLc : PMIOPort  Port=3  Side=Right
  CHM7a : PMIOPort  Port=4  Side=Right
  CHM7b : PMIOPort  Port=5  Side=Right
  CHM7c : PMIOPort  Port=6  Side=Right
  wires:
  Regulators2/1(Pm) -> LG3_2200 MVA/1
  Regulators4/2(Vf) -> LG4-2700 MVA/2
  Regulators4/1(Pm) -> LG4-2700 MVA/1
  Regulators3/2(Vf) -> LG31-200 MVA/2
  Regulators3/1(Pm) -> LG31-200 MVA/1
  Regulators2/2(Vf) -> LG3_2200 MVA/2
  LG3_2200 MVA/1 -> Regulators2/1(m)
  Regulators1/1(Pm) -> LG2_5500 MVA/1
  Regulators1/2(Vf) -> LG2_5500 MVA/2
  LG2_5500 MVA/1 -> Regulators1/1(m)
  LG31-200 MVA/1 -> Regulators3/1(m)
  LG4-2700 MVA/1 -> Regulators4/1(m)
  connections:
  LG2-NENI 3*279km/RConn1 -- "Cs NEM "/LConn1
  LG2-NENI 3*279km/RConn2 -- "Cs NEM "/LConn2
  LG2-NENI 3*279km/RConn3 -- "Cs NEM "/LConn3
  CHB-CHM 3*195km/RConn1 -- "Cs  CHMN "/LConn1
  CHB-CHM 3*195km/RConn2 -- "Cs  CHMN "/LConn2
  CHB-CHM 3*195km/RConn3 -- "Cs  CHMN "/LConn3
  Load Flow Bus2/LConn1 -- 2200 MVA 13.8 kV/735 kV/LConn1 -- LG3_2200 MVA/RConn1 -- 110 MW/LConn1
  2200 MVA 13.8 kV/735 kV/LConn2 -- LG3_2200 MVA/RConn2 -- 110 MW/LConn2
  2200 MVA 13.8 kV/735 kV/LConn3 -- LG3_2200 MVA/RConn3 -- 110 MW/LConn3
  Load Flow Bus1/LConn1 -- 200 MVA 13.8 kV/735 kV/LConn1 -- LG31-200 MVA/RConn1 -- 10 MW/LConn1
  200 MVA 13.8 kV/735 kV/LConn2 -- LG31-200 MVA/RConn2 -- 10 MW/LConn2
  200 MVA 13.8 kV/735 kV/LConn3 -- LG31-200 MVA/RConn3 -- 10 MW/LConn3
  Load Flow Bus6/LConn1 -- 2200 MVA 13.8 kV/735 kV/RConn1 -- 200 MVA 13.8 kV/735 kV/RConn1 -- LG3-LMO 104km/LConn1 -- LG3 660 Mvar/LConn1 -- LG2-LG3 155km/RConn1
  2200 MVA 13.8 kV/735 kV/RConn2 -- LG3 660 Mvar/LConn2 -- LG2-LG3 155km/RConn2 -- 200 MVA 13.8 kV/735 kV/RConn2 -- LG3-LMO 104km/LConn2
  LG3-LMO 104km/RConn1 -- LMO7/RConn1 -- LG4-LMO 3*118km/RConn1 -- LMO 330 Mvar/LConn1
  LG3-LMO 104km/RConn2 -- LMO7/RConn2 -- LG4-LMO 3*118km/RConn2 -- LMO 330 Mvar/LConn2
  LG3-LMO 104km/RConn3 -- LMO7/RConn3 -- LG4-LMO 3*118km/RConn3 -- LMO 330 Mvar/LConn3
  LG4-LMO 3*118km/LConn1 -- LG4 660 Mvar/LConn1 -- 2700 MVA 13.8 kV/735 kV/RConn1 -- Load Flow Bus12/LConn1
  LG4-LMO 3*118km/LConn2 -- 2700 MVA 13.8 kV/735 kV/RConn2 -- LG4 660 Mvar/LConn2
  LG4 660 Mvar/LConn3 -- 2700 MVA 13.8 kV/735 kV/RConn3 -- LG4-LMO 3*118km/LConn3
  Load Flow Bus3/LConn1 -- LG4-2700 MVA/RConn1 -- 2700 MVA 13.8 kV/735 kV/LConn1 -- 135 MW/LConn1
  LG4-2700 MVA/RConn2 -- 2700 MVA 13.8 kV/735 kV/LConn2 -- 135 MW/LConn2
  LG4-2700 MVA/RConn3 -- 2700 MVA 13.8 kV/735 kV/LConn3 -- 135 MW/LConn3
  Load Flow Bus4/LConn1 -- 5500 MVA 13.8 kV/735 kV/LConn1 -- LG2_5500 MVA/RConn1 -- 275 MW/LConn1
  5500 MVA 13.8 kV/735 kV/LConn2 -- LG2_5500 MVA/RConn2 -- 275 MW/LConn2
  LG2_5500 MVA/RConn3 -- 5500 MVA 13.8 kV/735 kV/LConn3 -- 275 MW/LConn3
  5500 MVA 13.8 kV/735 kV/RConn1 -- LG2-NENI 3*279km/LConn1 -- LG2-LG3 155km/LConn1 -- LG2 660 Mvar/LConn1 -- Load Flow Bus5/LConn1
  LG2-LG3 155km/LConn2 -- 5500 MVA 13.8 kV/735 kV/RConn2 -- LG2-NENI 3*279km/LConn2 -- LG2 660 Mvar/LConn2
  LG2-LG3 155km/LConn3 -- 5500 MVA 13.8 kV/735 kV/RConn3 -- LG2-NENI 3*279km/LConn3 -- LG2 660 Mvar/LConn3
  "Cs NEM "/RConn1 -- NEM-ALB7/LConn1 -- Cs ALB/RConn1
  "Cs NEM "/RConn2 -- NEM-ALB7/LConn2 -- Cs ALB/RConn2
  "Cs NEM "/RConn3 -- NEM-ALB7/LConn3 -- Cs ALB/RConn3
  LMO7/LConn1 -- LMO-ALB 3*218km/LConn1
  LMO7/LConn2 -- LMO-ALB 3*218km/LConn2
  Load Flow Bus7/LConn1 -- LMO7/LConn3 -- LMO-ALB 3*218km/LConn3
  Cs ALB/LConn1 -- LMO-ALB 3*218km/RConn1
  Cs ALB/LConn2 -- LMO-ALB 3*218km/RConn2
  Cs ALB/LConn3 -- LMO-ALB 3*218km/RConn3
  200 MVA 13.8 kV/735 kV/RConn3 -- LG3-LMO 104km/LConn3 -- LG3 660 Mvar/LConn3 -- LG2-LG3 155km/RConn3 -- 2200 MVA 13.8 kV/735 kV/RConn3
  Load Flow Bus8/LConn1 -- NEM-ABI 6*236/LConn1 -- NEM-ALB7/RConn1 -- NEM-ALB 1980 Mvar/LConn1
  NEM-ALB 1980 Mvar/LConn2 -- NEM-ALB7/RConn2 -- NEM-ABI 6*236/LConn2
  NEM-ALB 1980 Mvar/LConn3 -- NEM-ALB7/RConn3 -- NEM-ABI 6*236/LConn3
  NEM-ABI 6*236/RConn1 -- "Cs ABI+CHB "/LConn1
  NEM-ABI 6*236/RConn2 -- "Cs ABI+CHB "/LConn2
  NEM-ABI 6*236/RConn3 -- "Cs ABI+CHB "/LConn3
  "Cs ABI+CHB "/RConn1 -- ABI-CHB7/LConn1
  "Cs ABI+CHB "/RConn2 -- ABI-CHB7/LConn2
  "Cs ABI+CHB "/RConn3 -- ABI-CHB7/LConn3
  Load Flow Bus9/LConn1 -- ABI+CHB 1320 Mvar/LConn1 -- CHB-CHM 3*195km/LConn1 -- ABI-CHB 3*271km/LConn1 -- ABI-CHB7/RConn1
  ABI-CHB 3*271km/LConn2 -- ABI-CHB7/RConn2 -- ABI+CHB 1320 Mvar/LConn2 -- CHB-CHM 3*195km/LConn2
  ABI-CHB 3*271km/LConn3 -- ABI-CHB7/RConn3 -- ABI+CHB 1320 Mvar/LConn3 -- CHB-CHM 3*195km/LConn3
  ABI-CHB 3*271km/RConn1 -- "Cs LVDN "/LConn1
  ABI-CHB 3*271km/RConn2 -- "Cs LVDN "/LConn2
  ABI-CHB 3*271km/RConn3 -- "Cs LVDN "/LConn3
  "Cs LVDN "/RConn1 -- LVD7/LConn1
  "Cs LVDN "/RConn2 -- LVD7/LConn2
  "Cs LVDN "/RConn3 -- LVD7/LConn3
  "Cs LVDS "/LConn1 -- LVD 990 Mvar/LConn1 -- Load Flow Bus10/LConn1 -- LVD7/RConn1
  "Cs LVDS "/LConn2 -- LVD7/RConn2 -- LVD 990 Mvar/LConn2
  "Cs LVDS "/LConn3 -- LVD7/RConn3 -- LVD 990 Mvar/LConn3
  "Cs LVDS "/RConn1 -- LVD-MTL 3*260km/LConn1
  "Cs LVDS "/RConn2 -- LVD-MTL 3*260km/LConn2
  "Cs LVDS "/RConn3 -- LVD-MTL 3*260km/LConn3
  MTLa/RConn1 -- LVD-MTL 3*260km/RConn1
  MTLb/RConn1 -- LVD-MTL 3*260km/RConn2
  MTLc/RConn1 -- LVD-MTL 3*260km/RConn3
  "Cs  CHMN "/RConn1 -- CHM7/LConn1
  "Cs  CHMN "/RConn2 -- CHM7/LConn2
  "Cs  CHMN "/RConn3 -- CHM7/LConn3
  CHM 1320Mvar/LConn2 -- CHM7/RConn2 -- CHM7b/RConn1
  Load Flow Bus11/LConn1 -- CHM 1320Mvar/LConn3 -- CHM7c/RConn1 -- CHM7/RConn3
  CHM7a/RConn1 -- CHM 1320Mvar/LConn1 -- CHM7/RConn1
